simulink model "week1_problem1"  (R2020b)
settings: Solver=VariableStepAuto  StartTime=0.0  StopTime=10.0  RelTol=1e-3
values from neighbouring files (symbols this model uses):
  b = 50    [initialization_value.m]
  k1 = 50    [initialization_value.m]
  k12 = 25    [initialization_value.m]
  M1 = 100    [initialization_value.m]
  M2 = 50    [initialization_value.m]
settings Model: Creator=omkar  LastModifiedBy=omkar

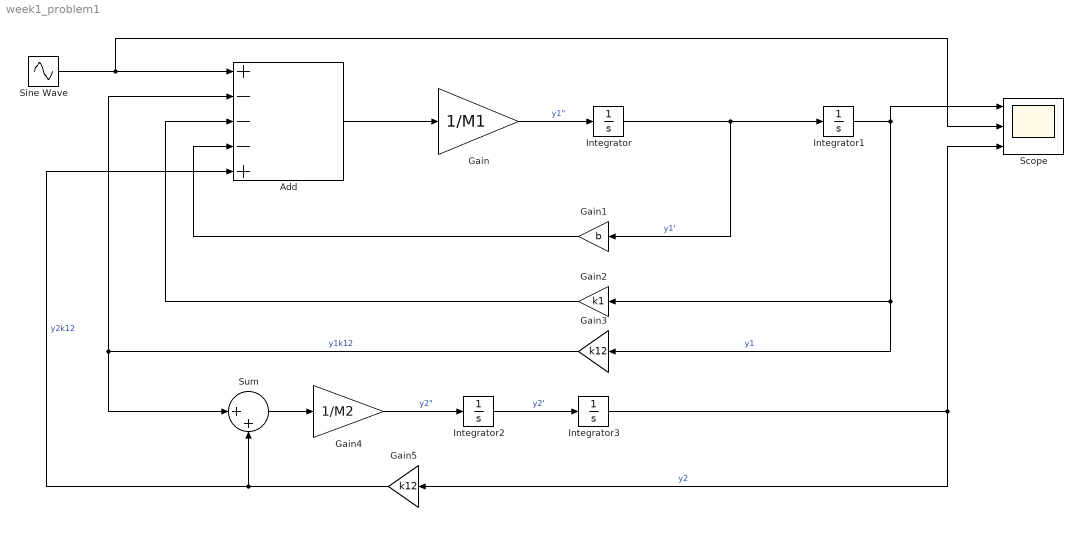
== system week1_problem1 ==
  Add : Sum  Inputs=+---+
  Gain : Gain  Gain=1/M1
  Gain1 : Gain  Gain=b
  Gain2 : Gain  Gain=k1
  Gain3 : Gain  Gain=k12
  Gain4 : Gain  Gain=1/M2
  Gain5 : Gain  Gain=k12
  Integrator{,1..3} (4 alike) : Integrator
  Scope : Scope  NumInputPorts=3
  Sine Wave : Sin  Frequency=10  SampleTime=0
  Sum : Sum  Inputs=|++
  wires:
  Sine Wave/1 -> Scope/2, Add/1
  Add/1 -> Gain/1
  Gain/1 -> Integrator/1  "y1''"
  Integrator/1 -> Gain1/1, Integrator1/1  "y1'"
  Gain1/1 -> Add/4
  Gain2/1 -> Add/3
  Integrator1/1 -> Gain3/1, Gain2/1, Scope/1  "y1"
  Gain3/1 -> Sum/1, Add/2  "y1k12"
  Sum/1 -> Gain4/1
  Gain4/1 -> Integrator2/1  "y2\""
  Integrator2/1 -> Integrator3/1  "y2'"
  Integrator3/1 -> Gain5/1, Scope/3  "y2"
  Gain5/1 -> Sum/2, Add/5  "y2k12"
